simulink model "full_bridge_R_load"  (Simulink 7.5)
settings: Solver=ode45  StartTime=0.0  StopTime=0.1  RelTol=1e-3
libraries: powerlib x13
settings Model: Creator=Manohar  LastModifiedBy=Manohar

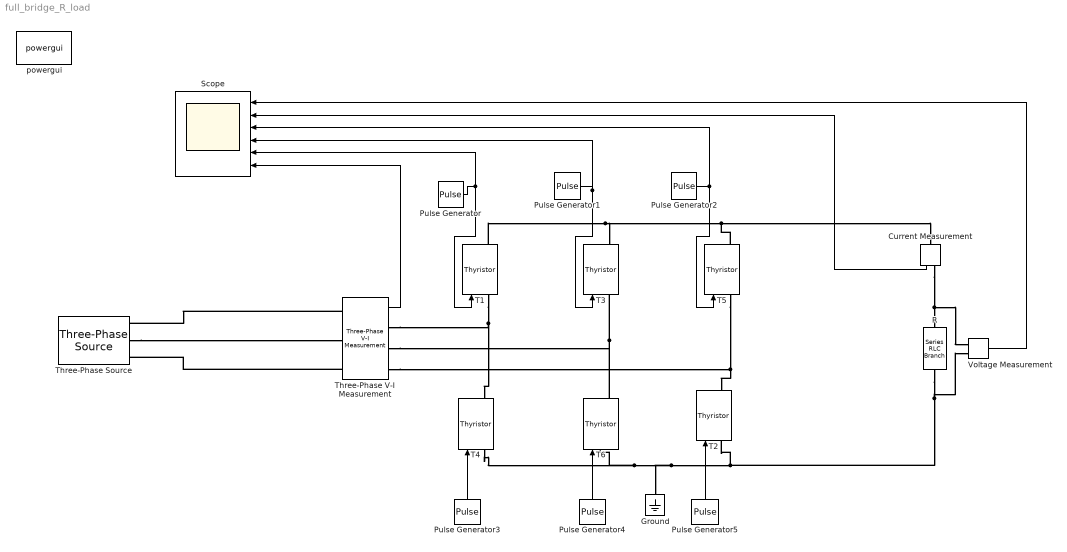
== system full_bridge_R_load ==
  Current Measurement : powerlib/Measurements/Current Measurement  DialogController=POWERSYS.PowerSysDialog  SystemSampleTime=-1  PhasorSimulation=off  OutputType=Complex  PSBequivalent=0
  Ground : powerlib/Elements/Ground  DialogController=POWERSYS.PowerSysDialog  PhysicalDomain=powersysdomain  SubClassName=unknown  LeftPortType=p1  RightPortType=p1  LConnTagsString=a
  Pulse Generator : DiscretePulseGenerator  PulseType=Time based  Amplitude=1  Period=0.02  PulseWidth=5  PhaseDelay=0.00666  SampleTime=1
  Pulse Generator1 : DiscretePulseGenerator  PulseType=Time based  Amplitude=1  Period=0.02  PulseWidth=5  PhaseDelay=.013333  SampleTime=1
  Pulse Generator2 : DiscretePulseGenerator  PulseType=Time based  Amplitude=1  Period=0.02  PulseWidth=5  PhaseDelay=0.02  SampleTime=1
  Pulse Generator3 : DiscretePulseGenerator  PulseType=Time based  Amplitude=1  Period=0.02  PulseWidth=5  PhaseDelay=0.0166666  SampleTime=1
  Pulse Generator4 : DiscretePulseGenerator  PulseType=Time based  Amplitude=1  Period=0.02  PulseWidth=5  PhaseDelay=0.02333  SampleTime=1
  Pulse Generator5 : DiscretePulseGenerator  PulseType=Time based  Amplitude=1  Period=0.02  PulseWidth=5  PhaseDelay=0.01  SampleTime=1
  R : powerlib/Elements/Series RLC Branch  DialogController=POWERSYS.PowerSysDialog  PhysicalDomain=powersysdomain  SubClassName=unknown  LeftPortType=p1  RightPortType=p1  LConnTagsString=__new0  RConnTagsString=__new0  BranchType=R  Resistance=100  Inductance=10  SetiL0=on  InitialCurrent=0  Capacitance=[]  Setx0=off  InitialVoltage=0  Measurements=None
  Scope : Scope  NumInputPorts=6
      settings: YMin=-5~-5~-5~-5~-5~-5  YMax=5~5~5~5~5~5
  T{1..6} (6 alike) : powerlib/Power Electronics/Thyristor  DialogController=POWERSYS.PowerSysDialog  SystemSampleTime=-1  Ron=0.001  Lon=0  Vf=0.8  IC=0  Rs=500  Cs=250e-9  Measurements=on
  Three-Phase V-I Measurement : powerlib/Measurements/Three-Phase V-I Measurement  DialogController=POWERSYS.PowerSysDialog  SystemSampleTime=-1  VoltageMeasurement=phase-to-ground  SetLabelV=off  LabelV=Vabc  Vpu=off  VpuLL=off  CurrentMeasurement=no  SetLabelI=off  LabelI=Iabc  Ipu=off  Pbase=100e6  Vbase=500e3  OutputType=Complex  PhasorSimulation=off  PSBequivalent=0
  Three-Phase Source : powerlib/Electrical Sources/Three-Phase Source  DialogController=POWERSYS.PowerSysDialog  SystemSampleTime=-1  Voltage=100  PhaseAngle=0  Frequency=50  InternalConnection=Yg  SpecifyImpedance=off  Resistance=0  Inductance=0  ShortCircuitLevel=100  BaseVoltage=25  XRratio=7
  Voltage Measurement : powerlib/Measurements/Voltage Measurement  DialogController=POWERSYS.PowerSysDialog  SystemSampleTime=-1  PhasorSimulation=off  OutputType=Complex  PSBequivalent=0
  powergui : powerlib/powergui  Priority=1  SystemSampleTime=-1  SimulationMode=Continuous  SampleTime=50e-6  frequency=60  SPID=off  DisableSnubberDevices=off  DisableRonSwitches=off  DisableVfSwitches=off  SwTol=0  Interpol=off  frequencyindice=50  echomessages=off  HookPort=off  DisplayEquations=off  FunctionMessages=off  EnableUseOfTLC=off  x0status=blocks  RestoreLinks=warning  ResistiveCurrentMeasurement=off  Ylog=off  Xlog=on  ShowGrid=off  save=off  variable=ZData  ZoomFFT=off  StartTime=0.0  cycles=1  DisplayStyle=1  FreqAxis=off  MaxFrequency=1000  frequencyindicesteady=1  display=off  methode=off
  wires:
  Pulse Generator/1 -> T1/1, Scope/5
  Pulse Generator1/1 -> T3/1, Scope/4
  Pulse Generator2/1 -> T5/1, Scope/3
  Voltage Measurement/1 -> Scope/1
  Current Measurement/1 -> Scope/2
  Three-Phase V-I Measurement/1 -> Scope/6
  Pulse Generator5/1 -> T2/1
  Pulse Generator4/1 -> T6/1
  Pulse Generator3/1 -> T4/1
  connections:
  T2/LConn1 -- T4/LConn1 -- T6/LConn1 -- Ground/LConn1 -- R/RConn1 -- Voltage Measurement/LConn2
  T4/RConn1 -- T1/LConn1 -- Three-Phase V-I Measurement/RConn1
  T6/RConn1 -- T3/LConn1 -- Three-Phase V-I Measurement/RConn2
  T5/LConn1 -- Three-Phase V-I Measurement/RConn3 -- T2/RConn1
  T5/RConn1 -- T1/RConn1 -- T3/RConn1 -- Current Measurement/LConn1
  Current Measurement/RConn1 -- R/LConn1 -- Voltage Measurement/LConn1
  Three-Phase V-I Measurement/LConn1 -- Three-Phase Source/RConn1
  Three-Phase V-I Measurement/LConn3 -- Three-Phase Source/RConn3
  Three-Phase Source/RConn2 -- Three-Phase V-I Measurement/LConn2
